simulink model "Copy_of_example_smc"  (R2020b)
settings: Solver=FixedStepAuto  StartTime=0.0  StopTime=10.0  FixedStep=0.001  RelTol=1e-3
libraries: fuzblock x7
settings Model: Creator=ShiningDanyang  LastModifiedBy=ShiningDanyang

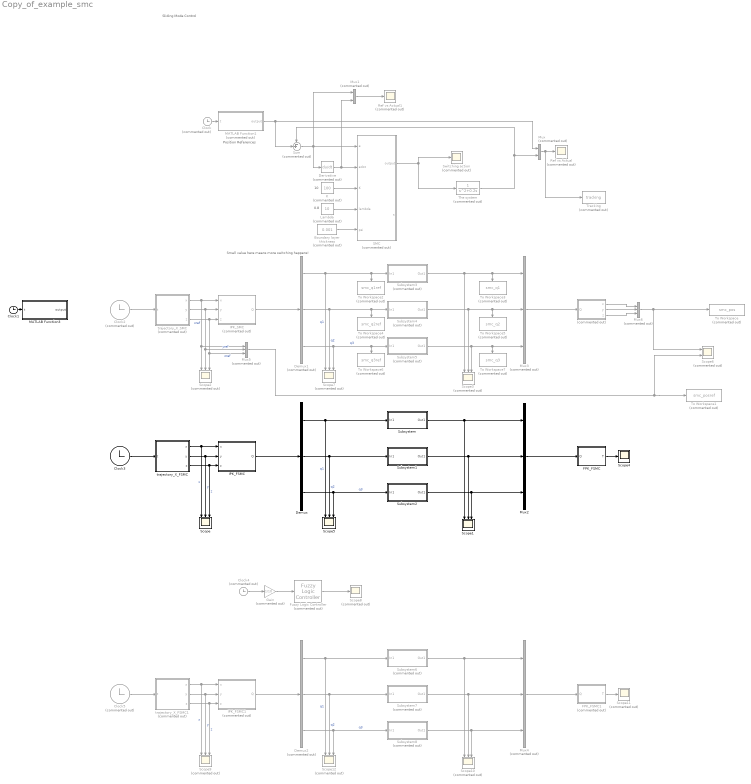
== system Copy_of_example_smc ==
  note: 10
  note: 0.8
  note: Sliding Mode Control
  note: Small value here means more switching happens!
  note: Position References
  " " : MATLAB Function  Commented=on  TreatAsAtomicUnit=on
  Boundary layer thickness : Constant  Commented=on  Value=0.001
  Clock{,2,4..5} (4 alike) : Clock  Commented=on
  Clock1 : Clock
  Clock3 : Clock
  Demux : Demux  Outputs=3
  Demux1 : Demux  Commented=on  Outputs=3
  Demux2 : Demux  Commented=on  Outputs=3
  Derivative : Derivative  Commented=on
  FPK_FSMC : MATLAB Function  TreatAsAtomicUnit=on
  FPK_FSMC1 : MATLAB Function  Commented=on  TreatAsAtomicUnit=on
  Fuzzy Logic Controller : fuzblock/Fuzzy Logic  Controller  Commented=on  FIS='fuzzy_example.fis'  OutputSampleNumber=101  DataType=double  FuzzifiedInputs=off  RuleFiringStrengths=off  RuleOutputs=off  AggregatedOutputs=off  SimulateUsing=Interpreted execution  OutOfRangeInputValueMessage=warning  NoRuleFiredMessage=warning  EmptyOutputFuzzySetMessage=warning
  Gain : Gain  Commented=on  Gain=1/10
  IPK_FSMC : MATLAB Function  TreatAsAtomicUnit=on
  IPK_FSMC1 : MATLAB Function  Commented=on  TreatAsAtomicUnit=on
  IPK_SMC : MATLAB Function  Commented=on  TreatAsAtomicUnit=on
  K : Constant  Commented=on  Value=100
  Lambda : Constant  Commented=on  Value=10
  MATLAB Function1 : MATLAB Function  Commented=on  TreatAsAtomicUnit=on
  MATLAB Function3 : MATLAB Function  TreatAsAtomicUnit=on
  Mux : Mux  Commented=on  Inputs=2
  Mux1 : Mux  Commented=on  Inputs=2
  Mux2 : Mux  Inputs=3
  Mux{3..6} (4 alike) : Mux  Commented=on  Inputs=3
  Ref vs Actual : Scope  Commented=on
  Ref vs Actual1 : Scope  Commented=on
  SMC : MATLAB Function  Commented=on  TreatAsAtomicUnit=on
  Scope : Scope  NumInputPorts=3
  Scope1 : Scope  NumInputPorts=3
  Scope{2..3,7,9..10,12} (6 alike) : Scope  Commented=on  NumInputPorts=3
  Scope11 : Scope  Commented=on
  Scope4 : Scope
  Scope5 : Scope  NumInputPorts=3
  Scope6 : Scope  Commented=on  NumInputPorts=2
  Scope8 : Scope  Commented=on
  Subsystem : Subsystem
  Subsystem1 : Subsystem
  Subsystem2 : Subsystem
  Subsystem3 : Subsystem  Commented=on
  Subsystem4 : Subsystem  Commented=on
  Subsystem5 : Subsystem  Commented=on
  Subsystem6 : Subsystem  Commented=on
  Subsystem7 : Subsystem  Commented=on
  Subsystem8 : Subsystem  Commented=on
  Sum : Sum  Commented=on  Inputs=-+|
  Switching action : Scope  Commented=on
  The system : TransferFcn  Commented=on  Denominator=[1 0.2 0]
  To Workspace : ToWorkspace  Commented=on  VariableName=smc_pos  SaveFormat=Timeseries  SampleTime=-1
  To Workspace1 : ToWorkspace  Commented=on  VariableName=smc_posref  SaveFormat=Timeseries  SampleTime=-1
  To Workspace2 : ToWorkspace  Commented=on  VariableName=smc_q1ref  SaveFormat=Timeseries  SampleTime=-1
  To Workspace3 : ToWorkspace  Commented=on  VariableName=smc_q1  SaveFormat=Timeseries  SampleTime=-1
  To Workspace4 : ToWorkspace  Commented=on  VariableName=smc_q2ref  SaveFormat=Timeseries  SampleTime=-1
  To Workspace5 : ToWorkspace  Commented=on  VariableName=smc_q2  SaveFormat=Timeseries  SampleTime=-1
  To Workspace6 : ToWorkspace  Commented=on  VariableName=smc_q3ref  SaveFormat=Timeseries  SampleTime=-1
  To Workspace7 : ToWorkspace  Commented=on  VariableName=smc_q3  SaveFormat=Timeseries  SampleTime=-1
  Tracking : ToWorkspace  Commented=on  VariableName=tracking  SampleTime=-1
  trajectory_X_FSMC : MATLAB Function  TreatAsAtomicUnit=on
  trajectory_X_FSMC1 : MATLAB Function  Commented=on  TreatAsAtomicUnit=on
  trajectory_X_SMC : MATLAB Function  Commented=on  TreatAsAtomicUnit=on
  wires:
  SMC/1(output) -> The system/1, Switching action/1
  MATLAB Function1/1(output) -> Mux/1, Sum/2
  Lambda/1 -> SMC/4(lambda)
  Clock/1 -> MATLAB Function1/1(t)
  Boundary layer thickness/1 -> SMC/5(psi)
  The system/1 -> Sum/1, Mux/2
  Sum/1 -> Mux1/1, SMC/1(e), Derivative/1
  K/1 -> SMC/3(K)
  Derivative/1 -> Mux1/2, SMC/2(edot)
  Mux1/1 -> Ref vs Actual1/1
  Mux/1 -> Tracking/1, Ref vs Actual/1
  Clock1/1 -> MATLAB Function3/1(t)
  Demux/1 -> Subsystem/1(In1), Scope5/1  "q1"
  Demux/2 -> Subsystem1/1(In1), Scope5/2  "q2"
  Demux/3 -> Subsystem2/1(In1), Scope5/3  "q3"
  FPK_FSMC/1(T) -> Scope4/1
  Subsystem/1(Out1) -> Mux2/1, Scope1/1
  Subsystem1/1(Out1) -> Mux2/2, Scope1/2
  Subsystem2/1(Out1) -> Mux2/3, Scope1/3
  Clock3/1 -> trajectory_X_FSMC/1(t)
  trajectory_X_FSMC/1(x) -> IPK_FSMC/1(x), Scope/1  "x"
  trajectory_X_FSMC/2(y) -> Scope/2, IPK_FSMC/2(y)  "y"
  trajectory_X_FSMC/3(z) -> Scope/3, IPK_FSMC/3(z)  "z"
  IPK_FSMC/1(Q) -> Demux/1
  Mux2/1 -> FPK_FSMC/1(Q)
  Mux3/1 -> " "/1(Q)
  IPK_SMC/1(Q) -> Demux1/1
  trajectory_X_SMC/2(y) -> Scope2/2, Mux5/2, IPK_SMC/2(y)  "yref"
  trajectory_X_SMC/3(z) -> Scope2/3, Mux5/3, IPK_SMC/3(z)  "zref"
  Subsystem4/1(Out1) -> Mux3/2, To Workspace5/1, Scope3/2
  Subsystem5/1(Out1) -> To Workspace7/1, Mux3/3, Scope3/3
  Demux1/3 -> To Workspace6/1, Subsystem5/1(In1), Scope7/3  "q3"
  Demux1/2 -> Subsystem4/1(In1), To Workspace4/1, Scope7/2  "q2"
  Demux1/1 -> Subsystem3/1(In1), To Workspace2/1, Scope7/1  "q1"
  Subsystem3/1(Out1) -> Mux3/1, To Workspace3/1, Scope3/1
  Clock2/1 -> trajectory_X_SMC/1(t)
  trajectory_X_SMC/1(x) -> IPK_SMC/1(x), Scope2/1, Mux5/1  "xref"
  Clock4/1 -> Gain/1
  Fuzzy Logic Controller/1 -> Scope8/1
  Gain/1 -> Fuzzy Logic Controller/1
  trajectory_X_FSMC1/3(z) -> Scope9/3, IPK_FSMC1/3(z)  "z"
  trajectory_X_FSMC1/1(x) -> IPK_FSMC1/1(x), Scope9/1  "x"
  Clock5/1 -> trajectory_X_FSMC1/1(t)
  trajectory_X_FSMC1/2(y) -> Scope9/2, IPK_FSMC1/2(y)  "y"
  Subsystem6/1(Out1) -> Mux4/1, Scope10/1
  Demux2/3 -> Subsystem8/1(In1), Scope12/3  "q3"
  Demux2/1 -> Subsystem6/1(In1), Scope12/1  "q1"
  IPK_FSMC1/1(Q) -> Demux2/1
  Demux2/2 -> Subsystem7/1(In1), Scope12/2  "q2"
  FPK_FSMC1/1(T) -> Scope11/1
  Subsystem8/1(Out1) -> Mux4/3, Scope10/3
  Mux4/1 -> FPK_FSMC1/1(Q)
  Subsystem7/1(Out1) -> Mux4/2, Scope10/2
  Mux5/1 -> To Workspace1/1, Scope6/2
  " "/2(y) -> Mux6/2
  " "/1(x) -> Mux6/1
  " "/3(z) -> Mux6/3
  Mux6/1 -> Scope6/1, To Workspace/1

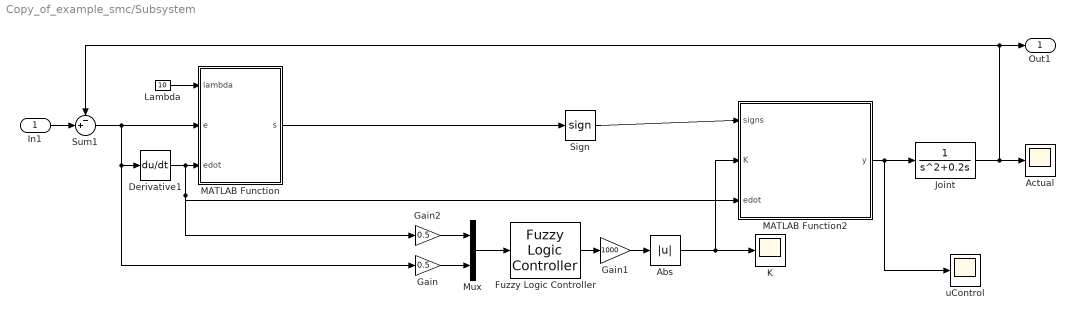
== system Copy_of_example_smc/Subsystem ==
  In1 : Inport
  Abs : Abs
  Actual : Scope
  Derivative1 : Derivative
  Fuzzy Logic Controller : fuzblock/Fuzzy Logic  Controller  FIS='fuzzy_example_nouse.fis'  OutputSampleNumber=101  DataType=double  FuzzifiedInputs=off  RuleFiringStrengths=off  RuleOutputs=off  AggregatedOutputs=off  SimulateUsing=Interpreted execution  OutOfRangeInputValueMessage=warning  NoRuleFiredMessage=warning  EmptyOutputFuzzySetMessage=warning
  Gain : Gain  Gain=0.5
  Gain1 : Gain  Gain=1000
  Gain2 : Gain  Gain=0.5
  Joint : TransferFcn  Denominator=[1 0.2 0]
  K : Scope
  Lambda : Constant  Value=10
  MATLAB Function : MATLAB Function  TreatAsAtomicUnit=on
  MATLAB Function2 : MATLAB Function  TreatAsAtomicUnit=on
  Mux : Mux  Inputs=2
  Sign : Signum
  Sum1 : Sum  Inputs=-+|
  uControl : Scope
  Out1 : Outport
  wires:
  MATLAB Function/1(s) -> Sign/1
  Lambda/1 -> MATLAB Function/1(lambda)
  Joint/1 -> Sum1/1, Out1/1, Actual/1
  MATLAB Function2/1(y) -> uControl/1, Joint/1
  Abs/1 -> K/1, MATLAB Function2/2(K)
  Fuzzy Logic Controller/1 -> Gain1/1
  Gain1/1 -> Abs/1
  Sum1/1 -> Gain/1, Derivative1/1, MATLAB Function/2(e)
  In1/1 -> Sum1/2
  Sign/1 -> MATLAB Function2/1(signs)
  Derivative1/1 -> MATLAB Function/3(edot), Gain2/1, MATLAB Function2/3(edot)
  Gain/1 -> Mux/2
  Gain2/1 -> Mux/1
  Mux/1 -> Fuzzy Logic Controller/1

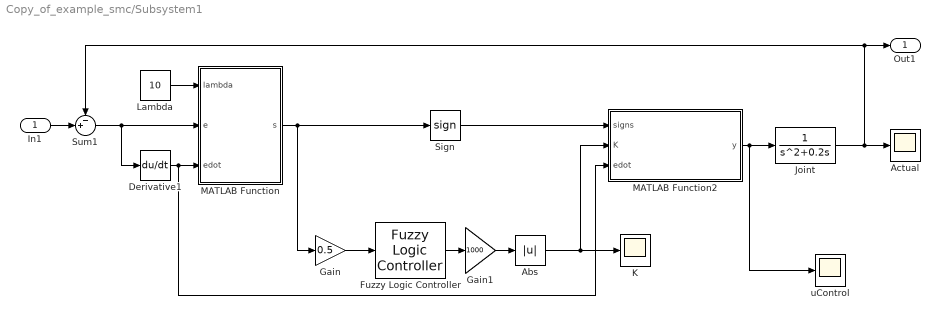
== system Copy_of_example_smc/Subsystem1 ==
  In1 : Inport
  Abs : Abs
  Actual : Scope
  Derivative1 : Derivative
  Fuzzy Logic Controller : fuzblock/Fuzzy Logic  Controller  FIS='fuzzy_example.fis'  OutputSampleNumber=101  DataType=double  FuzzifiedInputs=off  RuleFiringStrengths=off  RuleOutputs=off  AggregatedOutputs=off  SimulateUsing=Interpreted execution  OutOfRangeInputValueMessage=warning  NoRuleFiredMessage=warning  EmptyOutputFuzzySetMessage=warning
  Gain : Gain  Gain=0.5
  Gain1 : Gain  Gain=1000
  Joint : TransferFcn  Denominator=[1 0.2 0]
  K : Scope
  Lambda : Constant  Value=10
  MATLAB Function : MATLAB Function  TreatAsAtomicUnit=on
  MATLAB Function2 : MATLAB Function  TreatAsAtomicUnit=on
  Sign : Signum
  Sum1 : Sum  Inputs=-+|
  uControl : Scope
  Out1 : Outport
  wires:
  MATLAB Function/1(s) -> Gain/1, Sign/1
  Lambda/1 -> MATLAB Function/1(lambda)
  Joint/1 -> Actual/1, Sum1/1, Out1/1
  MATLAB Function2/1(y) -> uControl/1, Joint/1
  Abs/1 -> K/1, MATLAB Function2/2(K)
  Fuzzy Logic Controller/1 -> Gain1/1
  Gain1/1 -> Abs/1
  Sum1/1 -> Derivative1/1, MATLAB Function/2(e)
  Derivative1/1 -> MATLAB Function/3(edot), MATLAB Function2/3(edot)
  Gain/1 -> Fuzzy Logic Controller/1
  In1/1 -> Sum1/2
  Sign/1 -> MATLAB Function2/1(signs)

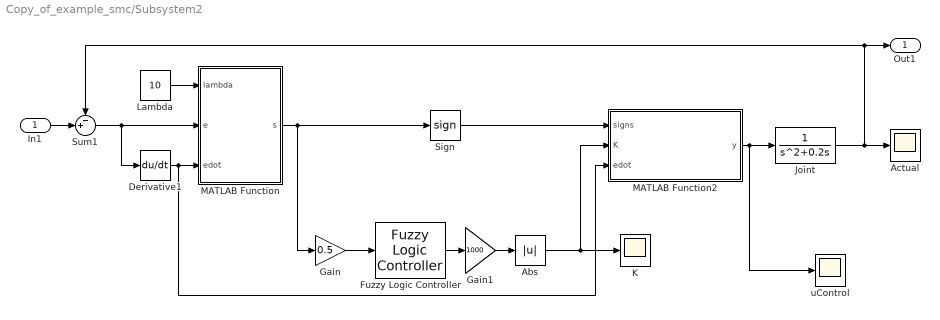
== system Copy_of_example_smc/Subsystem2 ==
  In1 : Inport
  Abs : Abs
  Actual : Scope
  Derivative1 : Derivative
  Fuzzy Logic Controller : fuzblock/Fuzzy Logic  Controller  FIS='fuzzy_example.fis'  OutputSampleNumber=101  DataType=double  FuzzifiedInputs=off  RuleFiringStrengths=off  RuleOutputs=off  AggregatedOutputs=off  SimulateUsing=Interpreted execution  OutOfRangeInputValueMessage=warning  NoRuleFiredMessage=warning  EmptyOutputFuzzySetMessage=warning
  Gain : Gain  Gain=0.5
  Gain1 : Gain  Gain=1000
  Joint : TransferFcn  Denominator=[1 0.2 0]
  K : Scope
  Lambda : Constant  Value=10
  MATLAB Function : MATLAB Function  TreatAsAtomicUnit=on
  MATLAB Function2 : MATLAB Function  TreatAsAtomicUnit=on
  Sign : Signum
  Sum1 : Sum  Inputs=-+|
  uControl : Scope
  Out1 : Outport
  wires:
  MATLAB Function/1(s) -> Gain/1, Sign/1
  Lambda/1 -> MATLAB Function/1(lambda)
  Joint/1 -> Actual/1, Sum1/1, Out1/1
  MATLAB Function2/1(y) -> uControl/1, Joint/1
  Abs/1 -> K/1, MATLAB Function2/2(K)
  Fuzzy Logic Controller/1 -> Gain1/1
  Gain1/1 -> Abs/1
  Sum1/1 -> Derivative1/1, MATLAB Function/2(e)
  Derivative1/1 -> MATLAB Function/3(edot), MATLAB Function2/3(edot)
  Gain/1 -> Fuzzy Logic Controller/1
  In1/1 -> Sum1/2
  Sign/1 -> MATLAB Function2/1(signs)

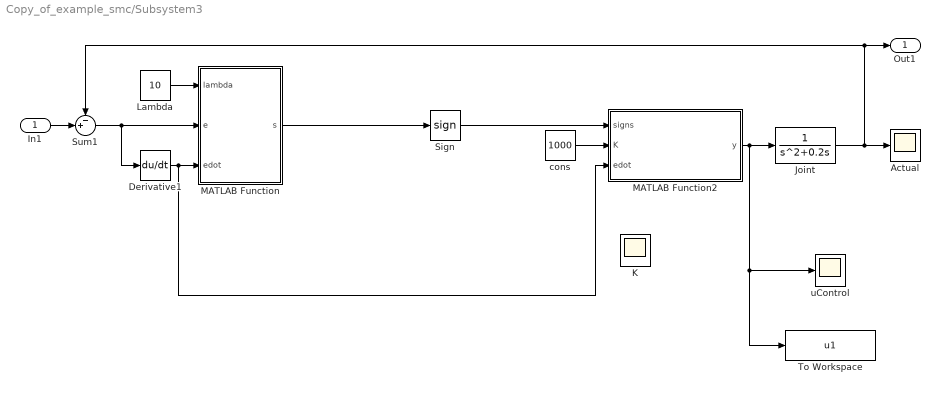
== system Copy_of_example_smc/Subsystem3 ==
  In1 : Inport
  Actual : Scope
  Derivative1 : Derivative
  Joint : TransferFcn  Denominator=[1 0.2 0]
  K : Scope
  Lambda : Constant  Value=10
  MATLAB Function : MATLAB Function  TreatAsAtomicUnit=on
  MATLAB Function2 : MATLAB Function  TreatAsAtomicUnit=on
  Sign : Signum
  Sum1 : Sum  Inputs=-+|
  To Workspace : ToWorkspace  VariableName=u1  SaveFormat=Timeseries  SampleTime=-1
  cons : Constant  Value=1000
  uControl : Scope
  Out1 : Outport
  wires:
  MATLAB Function/1(s) -> Sign/1
  Lambda/1 -> MATLAB Function/1(lambda)
  Joint/1 -> Actual/1, Sum1/1, Out1/1
  MATLAB Function2/1(y) -> To Workspace/1, uControl/1, Joint/1
  Sum1/1 -> Derivative1/1, MATLAB Function/2(e)
  Derivative1/1 -> MATLAB Function/3(edot), MATLAB Function2/3(edot)
  In1/1 -> Sum1/2
  Sign/1 -> MATLAB Function2/1(signs)
  cons/1 -> MATLAB Function2/2(K)

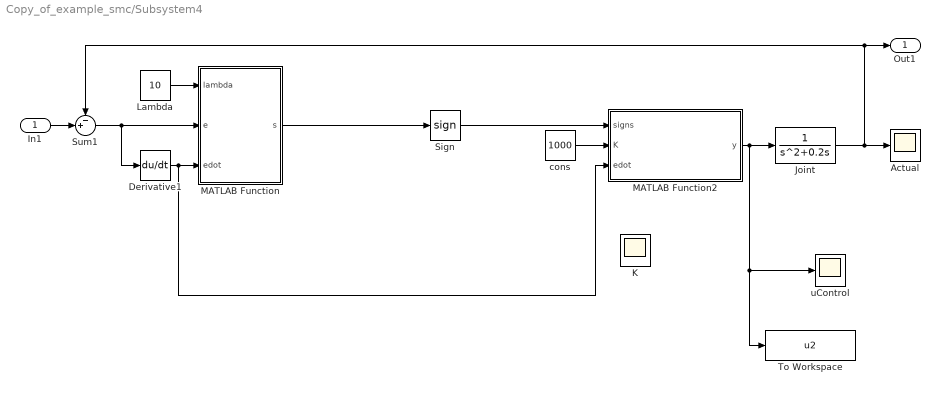
== system Copy_of_example_smc/Subsystem4 ==
  In1 : Inport
  Actual : Scope
  Derivative1 : Derivative
  Joint : TransferFcn  Denominator=[1 0.2 0]
  K : Scope
  Lambda : Constant  Value=10
  MATLAB Function : MATLAB Function  TreatAsAtomicUnit=on
  MATLAB Function2 : MATLAB Function  TreatAsAtomicUnit=on
  Sign : Signum
  Sum1 : Sum  Inputs=-+|
  To Workspace : ToWorkspace  VariableName=u2  SaveFormat=Timeseries  SampleTime=-1
  cons : Constant  Value=1000
  uControl : Scope
  Out1 : Outport
  wires:
  MATLAB Function/1(s) -> Sign/1
  Lambda/1 -> MATLAB Function/1(lambda)
  Joint/1 -> Actual/1, Sum1/1, Out1/1
  MATLAB Function2/1(y) -> To Workspace/1, uControl/1, Joint/1
  Sum1/1 -> Derivative1/1, MATLAB Function/2(e)
  Derivative1/1 -> MATLAB Function/3(edot), MATLAB Function2/3(edot)
  In1/1 -> Sum1/2
  Sign/1 -> MATLAB Function2/1(signs)
  cons/1 -> MATLAB Function2/2(K)

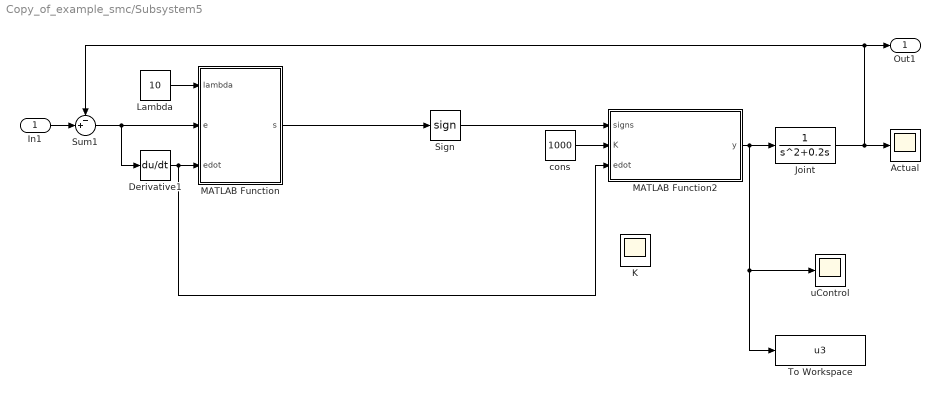
== system Copy_of_example_smc/Subsystem5 ==
  In1 : Inport
  Actual : Scope
  Derivative1 : Derivative
  Joint : TransferFcn  Denominator=[1 0.2 0]
  K : Scope
  Lambda : Constant  Value=10
  MATLAB Function : MATLAB Function  TreatAsAtomicUnit=on
  MATLAB Function2 : MATLAB Function  TreatAsAtomicUnit=on
  Sign : Signum
  Sum1 : Sum  Inputs=-+|
  To Workspace : ToWorkspace  VariableName=u3  SaveFormat=Timeseries  SampleTime=-1
  cons : Constant  Value=1000
  uControl : Scope
  Out1 : Outport
  wires:
  MATLAB Function/1(s) -> Sign/1
  Lambda/1 -> MATLAB Function/1(lambda)
  Joint/1 -> Actual/1, Sum1/1, Out1/1
  MATLAB Function2/1(y) -> To Workspace/1, uControl/1, Joint/1
  Sum1/1 -> Derivative1/1, MATLAB Function/2(e)
  Derivative1/1 -> MATLAB Function/3(edot), MATLAB Function2/3(edot)
  In1/1 -> Sum1/2
  Sign/1 -> MATLAB Function2/1(signs)
  cons/1 -> MATLAB Function2/2(K)

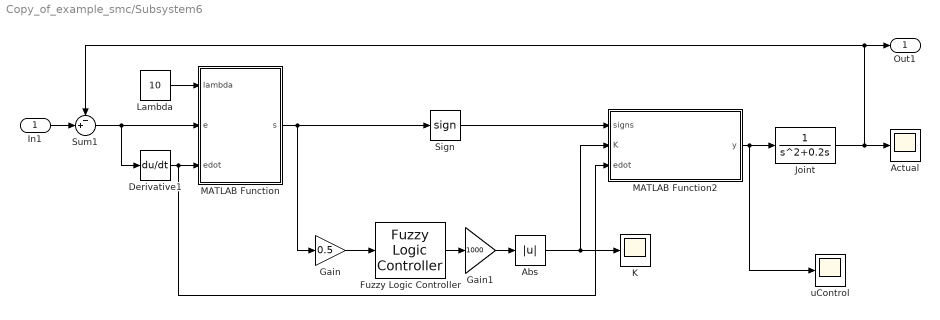
== system Copy_of_example_smc/Subsystem6 ==
  In1 : Inport
  Abs : Abs
  Actual : Scope
  Derivative1 : Derivative
  Fuzzy Logic Controller : fuzblock/Fuzzy Logic  Controller  FIS='fuzzy_example.fis'  OutputSampleNumber=101  DataType=double  FuzzifiedInputs=off  RuleFiringStrengths=off  RuleOutputs=off  AggregatedOutputs=off  SimulateUsing=Interpreted execution  OutOfRangeInputValueMessage=warning  NoRuleFiredMessage=warning  EmptyOutputFuzzySetMessage=warning
  Gain : Gain  Gain=0.5
  Gain1 : Gain  Gain=1000
  Joint : TransferFcn  Denominator=[1 0.2 0]
  K : Scope
  Lambda : Constant  Value=10
  MATLAB Function : MATLAB Function  TreatAsAtomicUnit=on
  MATLAB Function2 : MATLAB Function  TreatAsAtomicUnit=on
  Sign : Signum
  Sum1 : Sum  Inputs=-+|
  uControl : Scope
  Out1 : Outport
  wires:
  MATLAB Function/1(s) -> Gain/1, Sign/1
  Lambda/1 -> MATLAB Function/1(lambda)
  Joint/1 -> Actual/1, Sum1/1, Out1/1
  MATLAB Function2/1(y) -> uControl/1, Joint/1
  Abs/1 -> K/1, MATLAB Function2/2(K)
  Fuzzy Logic Controller/1 -> Gain1/1
  Gain1/1 -> Abs/1
  Sum1/1 -> Derivative1/1, MATLAB Function/2(e)
  Derivative1/1 -> MATLAB Function/3(edot), MATLAB Function2/3(edot)
  Gain/1 -> Fuzzy Logic Controller/1
  In1/1 -> Sum1/2
  Sign/1 -> MATLAB Function2/1(signs)

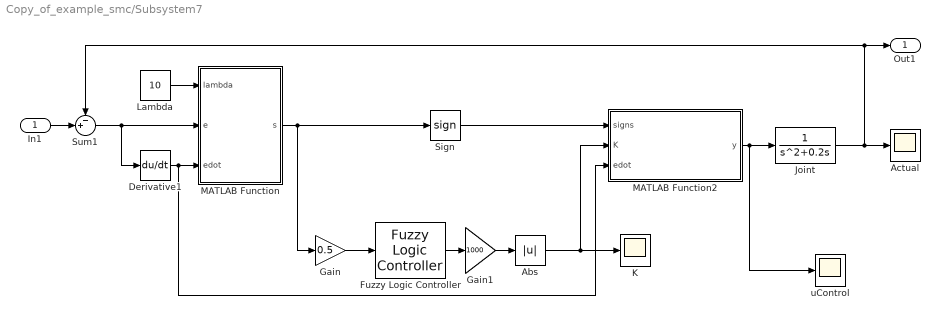
== system Copy_of_example_smc/Subsystem7 ==
  In1 : Inport
  Abs : Abs
  Actual : Scope
  Derivative1 : Derivative
  Fuzzy Logic Controller : fuzblock/Fuzzy Logic  Controller  FIS='fuzzy_example.fis'  OutputSampleNumber=101  DataType=double  FuzzifiedInputs=off  RuleFiringStrengths=off  RuleOutputs=off  AggregatedOutputs=off  SimulateUsing=Interpreted execution  OutOfRangeInputValueMessage=warning  NoRuleFiredMessage=warning  EmptyOutputFuzzySetMessage=warning
  Gain : Gain  Gain=0.5
  Gain1 : Gain  Gain=1000
  Joint : TransferFcn  Denominator=[1 0.2 0]
  K : Scope
  Lambda : Constant  Value=10
  MATLAB Function : MATLAB Function  TreatAsAtomicUnit=on
  MATLAB Function2 : MATLAB Function  TreatAsAtomicUnit=on
  Sign : Signum
  Sum1 : Sum  Inputs=-+|
  uControl : Scope
  Out1 : Outport
  wires:
  MATLAB Function/1(s) -> Gain/1, Sign/1
  Lambda/1 -> MATLAB Function/1(lambda)
  Joint/1 -> Actual/1, Sum1/1, Out1/1
  MATLAB Function2/1(y) -> uControl/1, Joint/1
  Abs/1 -> K/1, MATLAB Function2/2(K)
  Fuzzy Logic Controller/1 -> Gain1/1
  Gain1/1 -> Abs/1
  Sum1/1 -> Derivative1/1, MATLAB Function/2(e)
  Derivative1/1 -> MATLAB Function/3(edot), MATLAB Function2/3(edot)
  Gain/1 -> Fuzzy Logic Controller/1
  In1/1 -> Sum1/2
  Sign/1 -> MATLAB Function2/1(signs)

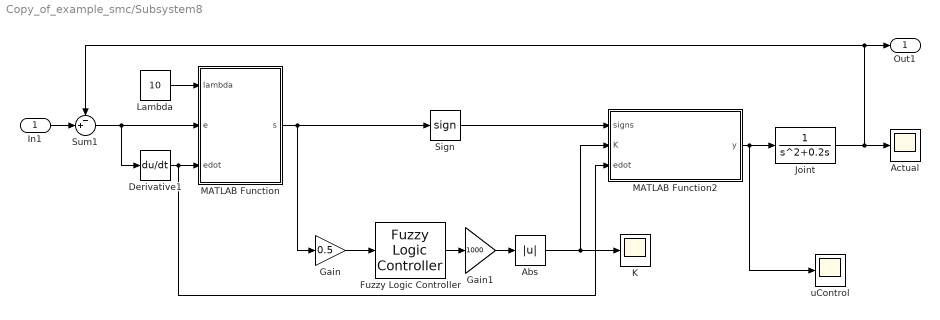
== system Copy_of_example_smc/Subsystem8 ==
  In1 : Inport
  Abs : Abs
  Actual : Scope
  Derivative1 : Derivative
  Fuzzy Logic Controller : fuzblock/Fuzzy Logic  Controller  FIS='fuzzy_example.fis'  OutputSampleNumber=101  DataType=double  FuzzifiedInputs=off  RuleFiringStrengths=off  RuleOutputs=off  AggregatedOutputs=off  SimulateUsing=Interpreted execution  OutOfRangeInputValueMessage=warning  NoRuleFiredMessage=warning  EmptyOutputFuzzySetMessage=warning
  Gain : Gain  Gain=0.5
  Gain1 : Gain  Gain=1000
  Joint : TransferFcn  Denominator=[1 0.2 0]
  K : Scope
  Lambda : Constant  Value=10
  MATLAB Function : MATLAB Function  TreatAsAtomicUnit=on
  MATLAB Function2 : MATLAB Function  TreatAsAtomicUnit=on
  Sign : Signum
  Sum1 : Sum  Inputs=-+|
  uControl : Scope
  Out1 : Outport
  wires:
  MATLAB Function/1(s) -> Gain/1, Sign/1
  Lambda/1 -> MATLAB Function/1(lambda)
  Joint/1 -> Actual/1, Sum1/1, Out1/1
  MATLAB Function2/1(y) -> uControl/1, Joint/1
  Abs/1 -> K/1, MATLAB Function2/2(K)
  Fuzzy Logic Controller/1 -> Gain1/1
  Gain1/1 -> Abs/1
  Sum1/1 -> Derivative1/1, MATLAB Function/2(e)
  Derivative1/1 -> MATLAB Function/3(edot), MATLAB Function2/3(edot)
  Gain/1 -> Fuzzy Logic Controller/1
  In1/1 -> Sum1/2
  Sign/1 -> MATLAB Function2/1(signs)

== matlab function Copy_of_example_smc/trajectory_X_FSMC ==
  data: x output; t input; y output; z output
function [x, y, z] = fcn(t)
tf = 1;
%start at [0; 0; -0.1585]
if(t<=2)
    x = 0;
    y = 0;
    z = -0.1585-t*0.0707;
    z = -0.3;
elseif(t<=4 && t>2)
    x = (t-2)/10;
    y = 0;
    z = -0.3;
    x = 0.2;
    y = 0;
    z = -0.3;
else
    x=0.2*cos(t-4);
    y=0.2*sin(t-4);
    z=-0.3;
end

== matlab function Copy_of_example_smc/  ==
  data: Q input; x output; y output; z output

% Nguyen Thinh 16CDT2
% Nguyen Quoc Thanh Giao 16CDT1
% 01/09/2019
%Ham tinh dong hoc thuan (FPK)
function [x,y,z]  = FPK_V2(Q)
%param
% Can 5 thong so 
% chieu dai canh tay L, chieu dai khau chap hanh cuoi l, chieu dai canh tam
% giac co dinh sB, chieu dai canh tam giac di dong sP.
% Thong so vi tri can tinh T=[x,y,z]
% Thong so goc quay Q=[q1,q2,q3]
%Chuyen tu do sang radian
% q1=(Q(1)*pi)/180;
% q2=(Q(2)*pi)/180;
% q3=(Q(3)*pi)/180;
q1 = Q(1);
q2 = Q(2);
q3 = Q(3);
%Cac thong so co ban cua delta robot
L=0.2; %Chieu dai canh tay lon
l=0.296; %Chieu dai canh tay nho
Sb = 0.2*sqrt(3); Sp = 0.05*sqrt(3);
% Thong so dung trong tinh toan
Wb=((sqrt(3)/6)*Sb);
Wp=(sqrt(3)/6)*Sp;
Ub=(sqrt(3)/3)*Sb;
Up=(sqrt(3)/3)*Sp;
% Dat cac bien a,b,c de dua he phuong trinh dong hoc thuan ve dang
% x^2 + (y+a+l.cos(q1))^2 + (z + l.sin(q1))^2 = l^2
% (X + b - (Sqrt(3)/2).l.cos(q2) )^2 + (Y + C - (1/2).l.cos(q2))^2 + ( Z + L.sin(q2) )^2 = l^2
% (X - b + (Sqrt(3)/2).l.cos(q3) )^2 + (Y + C - (1/2).l.cos(q3))^2 + ( Z + L.sin(q3) )^2 = l^2
%...........................
a=Wb-Up;
b=(Sp/2)-(sqrt(3)/2)*Wb;
c=Wp-Wb/2;
%...........................
% Dua he phuong trinh ve dang giao diem 3 mat cau
% Cac bien Xi,Yi,Zi voi i=1,2,3 la toa do cua tam 3 mat cau
% Cac bien Ri voi i=1,2,3 la ban kinh 3 mat cau
%.............................
X1=0;
Y1=-a-(L*cos(q1));
Z1=-L*sin(q1);
X2=(sqrt(3)/2)*L*cos(q2)-b;
Y2=((1/2)*L*cos(q2)) - c;
Z2= -L*sin(q2);
X3=-(sqrt(3)/2)*L*cos(q3)+b;
Y3=((1/2)*L*cos(q3)) - c;
Z3= -L*sin(q3);
R1=l;
R2=l;
R3=l;
%...........................
% Dua he giao diem 3 mat cau ve dang:
% a11.x + a12.y + a13.z = b1
% a21.x + a22.y + a23.z = b2
%...........................
a11=2*(X3-X1);
a12=2*(Y3-Y1);
a13=2*(Z3-Z1);
a21=2*(X3-X2);
a22=2*(Y3-Y2);
a23=2*(Z3-Z2);
b1=(R1^2)-(R3^2)-(X1^2)-(Y1^2)-(Z1^2)+(X3^2)+(Y3^2)+(Z3^2);
b2=(R2^2)-(R3^2)-(X2^2)-(Y2^2)-(Z2^2)+(X3^2)+(Y3^2)+(Z3^2);
%...........................
%Kiem tra cac diem ki di
if ((a13==0)||(a23==0))
% Giai theo phu luc B
% [A].[B]=[C] voi
% [A] = [m,n; p,q] ; [X]=[x,y] ; [C]= [k, t]
m = 2*(X3-X1);
n = 2*(Y3-Y1);
p = 2*(X3-X2);
q = 2*(Y3-Y2);
k = X3^2 + Y3^2 - X1^2 -Y1^2;
t = X3^2 + Y3^2 - X2^2 -Y2^2;
[A] = [m,n;p,q] ;
[B]=[;]; 
[C]= [k;t];
[B] = [A]\[C];
Zn=Z1;
x1=B(1);
x2=x1;
x=x1;
y1=B(2);
y2=y1;
y=y1;
% Giai phuong trinh bac 2 tim z
z1 = ((2*Zn) + ( sqrt((-2*Zn)^2 - 4*(Zn^2 - R1^2 + (x - X1)^2 + (y-Y1)^2 )) ))/2;
z2 = ((2*Zn) - ( sqrt((-2*Zn)^2 - 4*(Zn^2 - R1^2 + (x - X1)^2 + (y-Y1)^2 )) ))/2;
else
    % Rut x theo y ( x=f(y)= a4.y + a5 )
% Voi
a1=(a11/a13)-(a21/a23);
a2=(a12/a13)-(a22/a23);
a3=(b2/a23)-(b1/a13);
a4= -a2/a1;
a5= -a3/a1;

%........................
% Rut z theo y z = a6.y + a7
% Voi
a6= (-a21*a4-a22)/a23;
a7= (b2-a21*a5)/a23;
%....................
% Dua ve phuong trinh bac 2 theo y: y = a.y^2 + b.y + c
% Voi 
a=(a4^2)+(a6^2)+1;
b=2*a4*(a5-X1)-2*Y1+2*a6*(a7-Z1);
c=a5*(a5-2*X1)+a7*(a7-2*Z1)+X1^2+Y1^2+Z1^2-R1^2;
%.......................
% Tim nghiem y
y1=(-b+(sqrt(b*b-4*a*c)))/(2*a);
y2=(-b-(sqrt(b*b-4*a*c)))/(2*a);
%........................
% Tinh x,z theo y
x1=a4*y1+a5;
x2=a4*y2+a5;
z1=a6*y1+a7;
z2=a6*y2+a7;
%..........................
end
...........................
T1=[x1,y1,z1];
T2=[x2,y2,z2];
% Loai nghiem z duong 
if (z1<=0)
T=T1;    

else
 T=T2;   
end
x=T(1);
y=T(2);
z=T(3);

== matlab function Copy_of_example_smc/IPK_SMC ==
  data: x input; Q output; y input; z input
%% IPK: Ham tinh dong hoc nguoc robot delta.
%% Dau vao la vector vi tri [x,y,z], dau ra la vi tri
%% goc quay [q1,q2,q3]
function Q  = IPK(x,y,z)

 %% Khai bao cac hang so su dung
 Pi = 3.141;
 esilon = 10e-8;

 %% Khai bao thong so cua robot
Sb = 0.2*sqrt(3); Sp = 0.05*sqrt(3);
R=Sb/(2*sqrt(3)); r = Sp/(sqrt(3));
a=0.2; b=0.296; 
anpha1=-pi/2; anpha2=pi/6; anpha3=5*pi/6;
m1=0.42; m2=0.2; m3=0.75; IAy=m1*a*a/3; g=9.81;
L=a;
l=b;
 h = 0.131; %% chieu rong canh tay hinh binh hanh
 Ub = (sqrt(3) / 3) * Sb;
 Up = (sqrt(3) / 3) * Sp;
 Wb = (sqrt(3) / 6) * Sb;
 Wp = (sqrt(3) / 6) * Sp;

 %% Khai bao cac he so trong tinh toan
 a = (-(Up)+Wb);
 b = ((Sp / 2) - ((sqrt(3)) / 2)* Wb);
 c = (Wp - (Wb / 2));

 %% Ma tran chua thong so cua phuong trinh dong hoc nguoc
 E = zeros(1,3);
 F = zeros(1,3);
 G = zeros(1,3);
 Q = zeros(1,3);
 %% Phuong trinh dong hoc nguoc duoc dua ve dang
 %% Fi.Sin(Qi) + Ei.cos(Qi) + Gi = 0 voi:
 E(1) = (2 * L * (y + a));
 E(2) = (-L * (sqrt(3) * ((x + b)) + y + c));
 E(3) = (L * (sqrt(3) * ((x - b)) - y - c));
 F(1) = (2 * z * L);
 F(2) = 2 * z * L;
 F(3) = 2 * z * L;
 G(1) = x * x + y * y + z * z + a * a + L * L + 2 * y * a - l * l;
 G(2) = x * x + y * y + z * z + b * b + c * c + L * L + 2 * (x * b + y * c) - l * l;
 G(3) = x * x + y * y + z * z + b * b + c * c + L * L + 2 * (-(x * b) + y * c) - l * l;

 %% Kiem tra cac toa do vo nghiem.
 for i = 1:3
    if (( E(i)^2 + F(i)^2 - G(i)^2 ) < 0)

%          fprintf('Khong tim duoc nghiem dong co thu %d \n',i);
        disp('Khoong timf dduocwj nghieemj ddoongj cow thws');
        disp(i);
    else
        t1 = ( -F(i) + sqrt( E(i)^2 + F(i)^2 - G(i)^2 ))/( G(i) - E(i));
        t2 = ( -F(i) - sqrt( E(i)^2 + F(i)^2 - G(i)^2 ))/( G(i) - E(i));
        q11 = 2*atan(t1);
        q12 = 2*atan(t2);
        if abs(q11)>abs(q12)
%             Q(i) = (q12*180)/pi;
            Q(i) = q12;
        else
%             Q(i) = (q11*180)/pi;
            Q(i) = q11;
        end
     end
end

== matlab function Copy_of_example_smc/Subsystem3/MATLAB Function ==
  data: lambda input; s output; e input; edot input
function s = s_cal(lambda, e, edot)

s = lambda * e + edot;

== matlab function Copy_of_example_smc/Subsystem/MATLAB Function ==
  data: lambda input; s output; e input; edot input
function s = s_cal(lambda, e, edot)

s = lambda * e + edot;

== matlab function Copy_of_example_smc/FPK_FSMC ==
  data: Q input; T output

% Nguyen Thinh 16CDT2
% Nguyen Quoc Thanh Giao 16CDT1
% 01/09/2019
%Ham tinh dong hoc thuan (FPK)
function T  = FPK_V2(Q)
%param
% Can 5 thong so 
% chieu dai canh tay L, chieu dai khau chap hanh cuoi l, chieu dai canh tam
% giac co dinh sB, chieu dai canh tam giac di dong sP.
% Thong so vi tri can tinh T=[x,y,z]
% Thong so goc quay Q=[q1,q2,q3]
%Chuyen tu do sang radian
% q1=(Q(1)*pi)/180;
% q2=(Q(2)*pi)/180;
% q3=(Q(3)*pi)/180;
q1 = Q(1);
q2 = Q(2);
q3 = Q(3);
%Cac thong so co ban cua delta robot
L=0.2; %Chieu dai canh tay lon
l=0.296; %Chieu dai canh tay nho
Sb = 0.2*sqrt(3); Sp = 0.05*sqrt(3);
% Thong so dung trong tinh toan
Wb=((sqrt(3)/6)*Sb);
Wp=(sqrt(3)/6)*Sp;
Ub=(sqrt(3)/3)*Sb;
Up=(sqrt(3)/3)*Sp;
% Dat cac bien a,b,c de dua he phuong trinh dong hoc thuan ve dang
% x^2 + (y+a+l.cos(q1))^2 + (z + l.sin(q1))^2 = l^2
% (X + b - (Sqrt(3)/2).l.cos(q2) )^2 + (Y + C - (1/2).l.cos(q2))^2 + ( Z + L.sin(q2) )^2 = l^2
% (X - b + (Sqrt(3)/2).l.cos(q3) )^2 + (Y + C - (1/2).l.cos(q3))^2 + ( Z + L.sin(q3) )^2 = l^2
%...........................
a=Wb-Up;
b=(Sp/2)-(sqrt(3)/2)*Wb;
c=Wp-Wb/2;
%...........................
% Dua he phuong trinh ve dang giao diem 3 mat cau
% Cac bien Xi,Yi,Zi voi i=1,2,3 la toa do cua tam 3 mat cau
% Cac bien Ri voi i=1,2,3 la ban kinh 3 mat cau
%.............................
X1=0;
Y1=-a-(L*cos(q1));
Z1=-L*sin(q1);
X2=(sqrt(3)/2)*L*cos(q2)-b;
Y2=((1/2)*L*cos(q2)) - c;
Z2= -L*sin(q2);
X3=-(sqrt(3)/2)*L*cos(q3)+b;
Y3=((1/2)*L*cos(q3)) - c;
Z3= -L*sin(q3);
R1=l;
R2=l;
R3=l;
%...........................
% Dua he giao diem 3 mat cau ve dang:
% a11.x + a12.y + a13.z = b1
% a21.x + a22.y + a23.z = b2
%...........................
a11=2*(X3-X1);
a12=2*(Y3-Y1);
a13=2*(Z3-Z1);
a21=2*(X3-X2);
a22=2*(Y3-Y2);
a23=2*(Z3-Z2);
b1=(R1^2)-(R3^2)-(X1^2)-(Y1^2)-(Z1^2)+(X3^2)+(Y3^2)+(Z3^2);
b2=(R2^2)-(R3^2)-(X2^2)-(Y2^2)-(Z2^2)+(X3^2)+(Y3^2)+(Z3^2);
%...........................
%Kiem tra cac diem ki di
if ((a13==0)||(a23==0))
% Giai theo phu luc B
% [A].[B]=[C] voi
% [A] = [m,n; p,q] ; [X]=[x,y] ; [C]= [k, t]
m = 2*(X3-X1);
n = 2*(Y3-Y1);
p = 2*(X3-X2);
q = 2*(Y3-Y2);
k = X3^2 + Y3^2 - X1^2 -Y1^2;
t = X3^2 + Y3^2 - X2^2 -Y2^2;
[A] = [m,n;p,q] ;
[B]=[;]; 
[C]= [k;t];
[B] = [A]\[C];
Zn=Z1;
x1=B(1);
x2=x1;
x=x1;
y1=B(2);
y2=y1;
y=y1;
% Giai phuong trinh bac 2 tim z
z1 = ((2*Zn) + ( sqrt((-2*Zn)^2 - 4*(Zn^2 - R1^2 + (x - X1)^2 + (y-Y1)^2 )) ))/2;
z2 = ((2*Zn) - ( sqrt((-2*Zn)^2 - 4*(Zn^2 - R1^2 + (x - X1)^2 + (y-Y1)^2 )) ))/2;
else
    % Rut x theo y ( x=f(y)= a4.y + a5 )
% Voi
a1=(a11/a13)-(a21/a23);
a2=(a12/a13)-(a22/a23);
a3=(b2/a23)-(b1/a13);
a4= -a2/a1;
a5= -a3/a1;

%........................
% Rut z theo y z = a6.y + a7
% Voi
a6= (-a21*a4-a22)/a23;
a7= (b2-a21*a5)/a23;
%....................
% Dua ve phuong trinh bac 2 theo y: y = a.y^2 + b.y + c
% Voi 
a=(a4^2)+(a6^2)+1;
b=2*a4*(a5-X1)-2*Y1+2*a6*(a7-Z1);
c=a5*(a5-2*X1)+a7*(a7-2*Z1)+X1^2+Y1^2+Z1^2-R1^2;
%.......................
% Tim nghiem y
y1=(-b+(sqrt(b*b-4*a*c)))/(2*a);
y2=(-b-(sqrt(b*b-4*a*c)))/(2*a);
%........................
% Tinh x,z theo y
x1=a4*y1+a5;
x2=a4*y2+a5;
z1=a6*y1+a7;
z2=a6*y2+a7;
%..........................
end
...........................
T1=[x1,y1,z1];
T2=[x2,y2,z2];
% Loai nghiem z duong 
if (z1<=0)
T=T1;    
else
 T=T2;   
end

== matlab function Copy_of_example_smc/Subsystem3/MATLAB Function2 ==
  data: signs input; K input; edot input; y output
function y = output(signs,K,edot)
y = -(edot - K * signs);

== matlab function Copy_of_example_smc/Subsystem4/MATLAB Function ==
  data: lambda input; s output; e input; edot input
function s = s_cal(lambda, e, edot)

s = lambda * e + edot;

== matlab function Copy_of_example_smc/Subsystem4/MATLAB Function2 ==
  data: signs input; K input; edot input; y output
function y = output(signs,K,edot)
y = -(edot - K * signs);

== matlab function Copy_of_example_smc/Subsystem5/MATLAB Function ==
  data: lambda input; s output; e input; edot input
function s = s_cal(lambda, e, edot)

s = lambda * e + edot;

== matlab function Copy_of_example_smc/Subsystem5/MATLAB Function2 ==
  data: signs input; K input; edot input; y output
function y = output(signs,K,edot)
y = -(edot - K * signs);

== matlab function Copy_of_example_smc/trajectory_X_SMC ==
  data: x output; t input; y output; z output
function [x, y, z] = fcn(t)
tf = 1;
%start at [0; 0; -0.1585]
if(t<=2)
    x = 0;
    y = 0;
    z = -0.1585-t*0.0707;
    z = -0.3;
elseif(t<=4 && t>2)
    x = (t-2)/10;
    y = 0;
    z = -0.3;
    x = 0.2;
    y = 0;
    z = -0.3;
else
    x=0.2*cos(t-4);
    y=0.2*sin(t-4);
    z=-0.3;
end

== matlab function Copy_of_example_smc/FPK_FSMC1 ==
  data: Q input; T output

% Nguyen Thinh 16CDT2
% Nguyen Quoc Thanh Giao 16CDT1
% 01/09/2019
%Ham tinh dong hoc thuan (FPK)
function T  = FPK_V2(Q)
%param
% Can 5 thong so 
% chieu dai canh tay L, chieu dai khau chap hanh cuoi l, chieu dai canh tam
% giac co dinh sB, chieu dai canh tam giac di dong sP.
% Thong so vi tri can tinh T=[x,y,z]
% Thong so goc quay Q=[q1,q2,q3]
%Chuyen tu do sang radian
% q1=(Q(1)*pi)/180;
% q2=(Q(2)*pi)/180;
% q3=(Q(3)*pi)/180;
q1 = Q(1);
q2 = Q(2);
q3 = Q(3);
%Cac thong so co ban cua delta robot
L=0.2; %Chieu dai canh tay lon
l=0.296; %Chieu dai canh tay nho
Sb = 0.2*sqrt(3); Sp = 0.05*sqrt(3);
% Thong so dung trong tinh toan
Wb=((sqrt(3)/6)*Sb);
Wp=(sqrt(3)/6)*Sp;
Ub=(sqrt(3)/3)*Sb;
Up=(sqrt(3)/3)*Sp;
% Dat cac bien a,b,c de dua he phuong trinh dong hoc thuan ve dang
% x^2 + (y+a+l.cos(q1))^2 + (z + l.sin(q1))^2 = l^2
% (X + b - (Sqrt(3)/2).l.cos(q2) )^2 + (Y + C - (1/2).l.cos(q2))^2 + ( Z + L.sin(q2) )^2 = l^2
% (X - b + (Sqrt(3)/2).l.cos(q3) )^2 + (Y + C - (1/2).l.cos(q3))^2 + ( Z + L.sin(q3) )^2 = l^2
%...........................
a=Wb-Up;
b=(Sp/2)-(sqrt(3)/2)*Wb;
c=Wp-Wb/2;
%...........................
% Dua he phuong trinh ve dang giao diem 3 mat cau
% Cac bien Xi,Yi,Zi voi i=1,2,3 la toa do cua tam 3 mat cau
% Cac bien Ri voi i=1,2,3 la ban kinh 3 mat cau
%.............................
X1=0;
Y1=-a-(L*cos(q1));
Z1=-L*sin(q1);
X2=(sqrt(3)/2)*L*cos(q2)-b;
Y2=((1/2)*L*cos(q2)) - c;
Z2= -L*sin(q2);
X3=-(sqrt(3)/2)*L*cos(q3)+b;
Y3=((1/2)*L*cos(q3)) - c;
Z3= -L*sin(q3);
R1=l;
R2=l;
R3=l;
%...........................
% Dua he giao diem 3 mat cau ve dang:
% a11.x + a12.y + a13.z = b1
% a21.x + a22.y + a23.z = b2
%...........................
a11=2*(X3-X1);
a12=2*(Y3-Y1);
a13=2*(Z3-Z1);
a21=2*(X3-X2);
a22=2*(Y3-Y2);
a23=2*(Z3-Z2);
b1=(R1^2)-(R3^2)-(X1^2)-(Y1^2)-(Z1^2)+(X3^2)+(Y3^2)+(Z3^2);
b2=(R2^2)-(R3^2)-(X2^2)-(Y2^2)-(Z2^2)+(X3^2)+(Y3^2)+(Z3^2);
%...........................
%Kiem tra cac diem ki di
if ((a13==0)||(a23==0))
% Giai theo phu luc B
% [A].[B]=[C] voi
% [A] = [m,n; p,q] ; [X]=[x,y] ; [C]= [k, t]
m = 2*(X3-X1);
n = 2*(Y3-Y1);
p = 2*(X3-X2);
q = 2*(Y3-Y2);
k = X3^2 + Y3^2 - X1^2 -Y1^2;
t = X3^2 + Y3^2 - X2^2 -Y2^2;
[A] = [m,n;p,q] ;
[B]=[;]; 
[C]= [k;t];
[B] = [A]\[C];
Zn=Z1;
x1=B(1);
x2=x1;
x=x1;
y1=B(2);
y2=y1;
y=y1;
% Giai phuong trinh bac 2 tim z
z1 = ((2*Zn) + ( sqrt((-2*Zn)^2 - 4*(Zn^2 - R1^2 + (x - X1)^2 + (y-Y1)^2 )) ))/2;
z2 = ((2*Zn) - ( sqrt((-2*Zn)^2 - 4*(Zn^2 - R1^2 + (x - X1)^2 + (y-Y1)^2 )) ))/2;
else
    % Rut x theo y ( x=f(y)= a4.y + a5 )
% Voi
a1=(a11/a13)-(a21/a23);
a2=(a12/a13)-(a22/a23);
a3=(b2/a23)-(b1/a13);
a4= -a2/a1;
a5= -a3/a1;

%........................
% Rut z theo y z = a6.y + a7
% Voi
a6= (-a21*a4-a22)/a23;
a7= (b2-a21*a5)/a23;
%....................
% Dua ve phuong trinh bac 2 theo y: y = a.y^2 + b.y + c
% Voi 
a=(a4^2)+(a6^2)+1;
b=2*a4*(a5-X1)-2*Y1+2*a6*(a7-Z1);
c=a5*(a5-2*X1)+a7*(a7-2*Z1)+X1^2+Y1^2+Z1^2-R1^2;
%.......................
% Tim nghiem y
y1=(-b+(sqrt(b*b-4*a*c)))/(2*a);
y2=(-b-(sqrt(b*b-4*a*c)))/(2*a);
%........................
% Tinh x,z theo y
x1=a4*y1+a5;
x2=a4*y2+a5;
z1=a6*y1+a7;
z2=a6*y2+a7;
%..........................
end
...........................
T1=[x1,y1,z1];
T2=[x2,y2,z2];
% Loai nghiem z duong 
if (z1<=0)
T=T1;    
else
 T=T2;   
end

== matlab function Copy_of_example_smc/IPK_FSMC1 ==
  data: x input; Q output; y input; z input
%% IPK: Ham tinh dong hoc nguoc robot delta.
%% Dau vao la vector vi tri [x,y,z], dau ra la vi tri
%% goc quay [q1,q2,q3]
function Q  = IPK(x,y,z)

 %% Khai bao cac hang so su dung
 Pi = 3.141;
 esilon = 10e-8;

 %% Khai bao thong so cua robot
Sb = 0.2*sqrt(3); Sp = 0.05*sqrt(3);
R=Sb/(2*sqrt(3)); r = Sp/(sqrt(3));
a=0.2; b=0.296; 
anpha1=-pi/2; anpha2=pi/6; anpha3=5*pi/6;
m1=0.42; m2=0.2; m3=0.75; IAy=m1*a*a/3; g=9.81;
L=a;
l=b;
 h = 0.131; %% chieu rong canh tay hinh binh hanh
 Ub = (sqrt(3) / 3) * Sb;
 Up = (sqrt(3) / 3) * Sp;
 Wb = (sqrt(3) / 6) * Sb;
 Wp = (sqrt(3) / 6) * Sp;

 %% Khai bao cac he so trong tinh toan
 a = (-(Up)+Wb);
 b = ((Sp / 2) - ((sqrt(3)) / 2)* Wb);
 c = (Wp - (Wb / 2));

 %% Ma tran chua thong so cua phuong trinh dong hoc nguoc
 E = zeros(1,3);
 F = zeros(1,3);
 G = zeros(1,3);
 Q = zeros(1,3);
 %% Phuong trinh dong hoc nguoc duoc dua ve dang
 %% Fi.Sin(Qi) + Ei.cos(Qi) + Gi = 0 voi:
 E(1) = (2 * L * (y + a));
 E(2) = (-L * (sqrt(3) * ((x + b)) + y + c));
 E(3) = (L * (sqrt(3) * ((x - b)) - y - c));
 F(1) = (2 * z * L);
 F(2) = 2 * z * L;
 F(3) = 2 * z * L;
 G(1) = x * x + y * y + z * z + a * a + L * L + 2 * y * a - l * l;
 G(2) = x * x + y * y + z * z + b * b + c * c + L * L + 2 * (x * b + y * c) - l * l;
 G(3) = x * x + y * y + z * z + b * b + c * c + L * L + 2 * (-(x * b) + y * c) - l * l;

 %% Kiem tra cac toa do vo nghiem.
 for i = 1:3
    if (( E(i)^2 + F(i)^2 - G(i)^2 ) < 0)

%          fprintf('Khong tim duoc nghiem dong co thu %d \n',i);
        disp('Khoong timf dduocwj nghieemj ddoongj cow thws');
        disp(i);
    else
        t1 = ( -F(i) + sqrt( E(i)^2 + F(i)^2 - G(i)^2 ))/( G(i) - E(i));
        t2 = ( -F(i) - sqrt( E(i)^2 + F(i)^2 - G(i)^2 ))/( G(i) - E(i));
        q11 = 2*atan(t1);
        q12 = 2*atan(t2);
        if abs(q11)>abs(q12)
%             Q(i) = (q12*180)/pi;
            Q(i) = q12;
        else
%             Q(i) = (q11*180)/pi;
            Q(i) = q11;
        end
     end
end

== matlab function Copy_of_example_smc/Subsystem6/MATLAB Function ==
  data: lambda input; s output; e input; edot input
function s = s_cal(lambda, e, edot)

s = lambda * e + edot;

== matlab function Copy_of_example_smc/SMC ==
  data: e input; output output; edot input; K input; lambda input; psi input; s output
function [output, s]= smc(e, edot, K, lambda, psi)
%#codegen

    s = lambda * e + edot;
        
    if (abs(s) > psi)    
        sat_s = sign(s);
    else
        sat_s = s/psi;
    end
    
    output = -(edot - K * sat_s);

end

== matlab function Copy_of_example_smc/Subsystem6/MATLAB Function2 ==
  data: signs input; K input; edot input; y output
function y = output(signs,K,edot)
y = -(edot - K * signs);

== matlab function Copy_of_example_smc/Subsystem7/MATLAB Function ==
  data: lambda input; s output; e input; edot input
function s = s_cal(lambda, e, edot)

s = lambda * e + edot;

== matlab function Copy_of_example_smc/Subsystem7/MATLAB Function2 ==
  data: signs input; K input; edot input; y output
function y = output(signs,K,edot)
y = -(edot - K * signs);

== matlab function Copy_of_example_smc/Subsystem8/MATLAB Function ==
  data: lambda input; s output; e input; edot input
function s = s_cal(lambda, e, edot)

s = lambda * e + edot;

== matlab function Copy_of_example_smc/Subsystem8/MATLAB Function2 ==
  data: signs input; K input; edot input; y output
function y = output(signs,K,edot)
y = -(edot - K * signs);

== matlab function Copy_of_example_smc/trajectory_X_FSMC1 ==
  data: x output; t input; y output; z output
function [x, y, z] = fcn(t)
tf = 1;
%start at [0; 0; -0.1585]
if(t<=2)
    x = 0;
    y = 0;
    z = -0.1585-t*0.0707;
    z = -0.3;
elseif(t<=4 && t>2)
    x = (t-2)/10;
    y = 0;
    z = -0.3;
    x = 0.2;
    y = 0;
    z = -0.3;
else
    x=0.2*cos(t-4);
    y=0.2*sin(t-4);
    z=-0.3;
end

== matlab function Copy_of_example_smc/Subsystem/MATLAB Function2 ==
  data: signs input; K input; edot input; y output
function y = output(signs,K,edot)
y = -(edot - K * signs);

== matlab function Copy_of_example_smc/MATLAB Function1 ==
  data: t input; output output
function output = generate_input(t)
%#codegen

    output = -pi/2+52.5/180*pi*(1-cos(1.26*t));
end

== matlab function Copy_of_example_smc/MATLAB Function3 ==
  data: t input; output output
function output = generate_input(t)
%#codegen

    output = -pi/2+52.5/180*pi*(1-cos(1.26*t));
end

== matlab function Copy_of_example_smc/IPK_FSMC ==
  data: x input; Q output; y input; z input
%% IPK: Ham tinh dong hoc nguoc robot delta.
%% Dau vao la vector vi tri [x,y,z], dau ra la vi tri
%% goc quay [q1,q2,q3]
function Q  = IPK(x,y,z)

 %% Khai bao cac hang so su dung
 Pi = 3.141;
 esilon = 10e-8;

 %% Khai bao thong so cua robot
Sb = 0.2*sqrt(3); Sp = 0.05*sqrt(3);
R=Sb/(2*sqrt(3)); r = Sp/(sqrt(3));
a=0.2; b=0.296; 
anpha1=-pi/2; anpha2=pi/6; anpha3=5*pi/6;
m1=0.42; m2=0.2; m3=0.75; IAy=m1*a*a/3; g=9.81;
L=a;
l=b;
 h = 0.131; %% chieu rong canh tay hinh binh hanh
 Ub = (sqrt(3) / 3) * Sb;
 Up = (sqrt(3) / 3) * Sp;
 Wb = (sqrt(3) / 6) * Sb;
 Wp = (sqrt(3) / 6) * Sp;

 %% Khai bao cac he so trong tinh toan
 a = (-(Up)+Wb);
 b = ((Sp / 2) - ((sqrt(3)) / 2)* Wb);
 c = (Wp - (Wb / 2));

 %% Ma tran chua thong so cua phuong trinh dong hoc nguoc
 E = zeros(1,3);
 F = zeros(1,3);
 G = zeros(1,3);
 Q = zeros(1,3);
 %% Phuong trinh dong hoc nguoc duoc dua ve dang
 %% Fi.Sin(Qi) + Ei.cos(Qi) + Gi = 0 voi:
 E(1) = (2 * L * (y + a));
 E(2) = (-L * (sqrt(3) * ((x + b)) + y + c));
 E(3) = (L * (sqrt(3) * ((x - b)) - y - c));
 F(1) = (2 * z * L);
 F(2) = 2 * z * L;
 F(3) = 2 * z * L;
 G(1) = x * x + y * y + z * z + a * a + L * L + 2 * y * a - l * l;
 G(2) = x * x + y * y + z * z + b * b + c * c + L * L + 2 * (x * b + y * c) - l * l;
 G(3) = x * x + y * y + z * z + b * b + c * c + L * L + 2 * (-(x * b) + y * c) - l * l;

 %% Kiem tra cac toa do vo nghiem.
 for i = 1:3
    if (( E(i)^2 + F(i)^2 - G(i)^2 ) < 0)

%          fprintf('Khong tim duoc nghiem dong co thu %d \n',i);
        disp('Khoong timf dduocwj nghieemj ddoongj cow thws');
        disp(i);
    else
        t1 = ( -F(i) + sqrt( E(i)^2 + F(i)^2 - G(i)^2 ))/( G(i) - E(i));
        t2 = ( -F(i) - sqrt( E(i)^2 + F(i)^2 - G(i)^2 ))/( G(i) - E(i));
        q11 = 2*atan(t1);
        q12 = 2*atan(t2);
        if abs(q11)>abs(q12)
%             Q(i) = (q12*180)/pi;
            Q(i) = q12;
        else
%             Q(i) = (q11*180)/pi;
            Q(i) = q11;
        end
     end
end

== matlab function Copy_of_example_smc/Subsystem1/MATLAB Function ==
  data: lambda input; s output; e input; edot input
function s = s_cal(lambda, e, edot)

s = lambda * e + edot;

== matlab function Copy_of_example_smc/Subsystem1/MATLAB Function2 ==
  data: signs input; K input; edot input; y output
function y = output(signs,K,edot)
y = -(edot - K * signs);

== matlab function Copy_of_example_smc/Subsystem2/MATLAB Function ==
  data: lambda input; s output; e input; edot input
function s = s_cal(lambda, e, edot)

s = lambda * e + edot;

== matlab function Copy_of_example_smc/Subsystem2/MATLAB Function2 ==
  data: signs input; K input; edot input; y output
function y = output(signs,K,edot)
y = -(edot - K * signs);
